simulink model "Smart_Grid_2"  (R2024b)
settings: Solver=FixedStepAuto  StartTime=0.0  StopTime=0.5  FixedStep=1e-5  RelTol=1e-3
undefined symbols (not defined in the file): Ion, Lithium
libraries: spsSeriesRLCBranchLib x76, spsRMSLib x65, spsIGBTDiodeLib x41, eeGeneralControl x36, slpidlib x34, spsThreePhaseVIMeasurementLib x32, spsVoltageMeasurementLib x18, simulink x16, spsCurrentMeasurementLib x15, spsThreePhaseBreakerLib x12, spsAlphaBetaZerotodq0Lib x12, spsPower3phPhasorLib x10
(part 7 of 8)

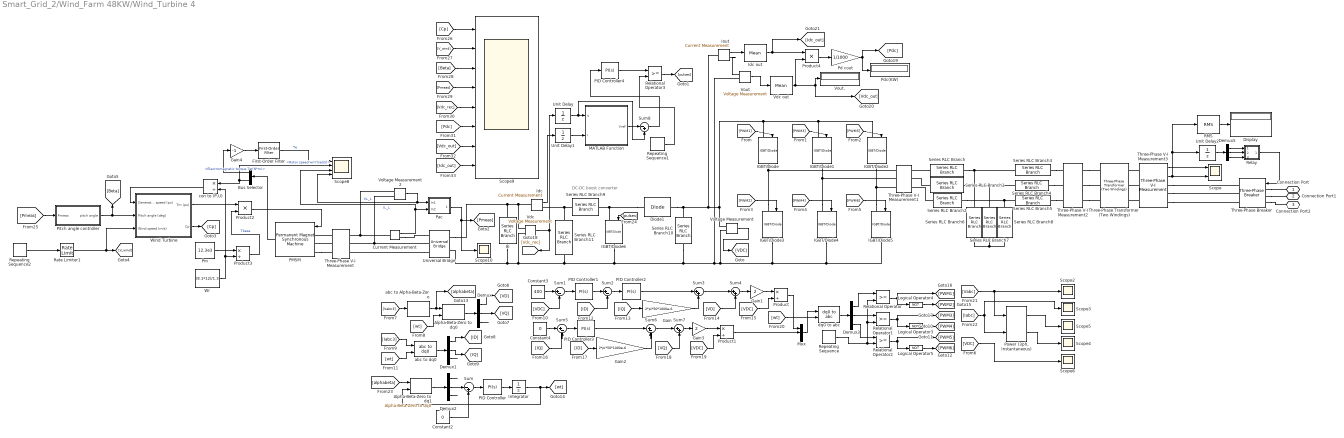
== system Smart_Grid_2/Wind_Farm 48KW/Wind_Turbine 4 ==
  note: DC-DC boost converter
  Alpha-Beta-Zero to dq0 : spsAlphaBetaZerotodq0Lib/Alpha-Beta-Zero to dq0  Alignment=90 degrees behind phase A axis
  Alpha-Beta-Zero to dq1 : spsAlphaBetaZerotodq0Lib/Alpha-Beta-Zero to dq0  Alignment=90 degrees behind phase A axis
  Bus Selector : BusSelector  OutputSignals=Electromagnetic torque Te (N*m),Rotor speed wm (rad/s)
  Ci : spsSeriesRLCBranchLib/Series RLC Branch  LConnTagsString=__new0  RConnTagsString=__new0  BranchType=RC  Resistance=0.005  Inductance=1e-3  SetiL0=off  InitialCurrent=0  Capacitance=500e-6  Setx0=off  InitialVoltage=0  Measurements=None
  Constant2 : Constant  Value=0
  Constant3 : Constant  Value=400
  Constant4 : Constant  Value=0
  Current Measurement : spsCurrentMeasurementLib/Current Measurement  PhasorSimulation=off  OutputType=Complex  PSBequivalent=0
  Demux{,1..3,5} (5 alike) : Demux  Outputs=3
  Diode1 : spsDiodeLib/Diode  Ron=0.001  Lon=0  Vf=0.8  IC=0  UseSnubber=0  Rs=500  Cs=250e-9  Measurements=off
  Display : Display
  First-Order Filter : spsFirstOrderFilterLib/First-Order Filter  FilterType=Lowpass  Tc=10e-3  Ts=50e-6  Initialize=on  Vac_Init=[0, 0, 50]  Vdc_Init=0  PlotResponse=off  FreqRange="[0,  200,  1]"
  Gain : Gain  Gain=2*pi*50*1000e-6
  Gain1 : Gain  Gain=2
  Gain2 : Gain  Gain=2*pi*50*1000e-6
  Gain3 : Gain  Gain=2
  Gain4 : Gain  Gain=-1
  IGBT/Diode{,1..6} (7 alike) : spsIGBTDiodeLib/IGBT//Diode  Ron=1e-3  Rs=1e5  Cs=inf  Measurements=off
  Idc : spsCurrentMeasurementLib/Current Measurement  PhasorSimulation=off  OutputType=Complex  PSBequivalent=0
  Idc out : spsMeanLib/Mean  Freq=50  Vinit=0  Ts=50e-6
  Integrator : Integrator
  Iout : spsCurrentMeasurementLib/Current Measurement  PhasorSimulation=off  OutputType=Complex  PSBequivalent=0
  Logical Operator3 : Logic  Operator=NOT  AllPortsSameDT=off  OutDataTypeStr=boolean
  Logical Operator4 : Logic  Operator=NOT  AllPortsSameDT=off  OutDataTypeStr=boolean
  Logical Operator5 : Logic  Operator=NOT  AllPortsSameDT=off  OutDataTypeStr=boolean
  MATLAB Function : MATLAB Function  TreatAsAtomicUnit=on
  Mux : Mux  Inputs=3
  PID Controller : slpidlib/PID Controller  Controller=PI  Form=Parallel  TimeDomain=Continuous-time  UseExternalTs=off  SampleTime=-1  IntegratorMethod=Forward Euler  FilterMethod=Forward Euler  ControllerParametersSource=internal  P=10  I=50000  UseKiTs=off  D=0  UseExternalDerivativeSource=off  N=100  UseFilter=on  TunerSelectOption=Transfer Function Based (PID Tuner App)  InitialConditionSource=internal  InitialConditionForIntegrator=0  InitialConditionForFilter=0  DifferentiatorICPrevScaledInput=0  ExternalReset=none  TrackingMode=off  Kt=1  LimitOutput=off  SatLimitsSource=internal  UpperSaturationLimit=inf  LowerSaturationLimit=-inf  LinearizeAsGain=on  AntiWindupMode=none  Kb=1  LimitIntegrator=off  UpperIntegratorSaturationLimit=inf  LowerIntegratorSaturationLimit=-inf  POutMin=[]  POutMax=[]  IOutMin=[]  IOutMax=[]  DOutMin=[]  DOutMax=[]  NOutMin=[]  NOutMax=[]  SumOutMin=[]  SumOutMax=[]  SaturationOutMin=[]  SaturationOutMax=[]  PParamMin=[]  PParamMax=[]  IParamMin=[]  IParamMax=[]  DParamMin=[]  DParamMax=[]  NParamMin=[]  NParamMax=[]  KbParamMin=[]  KbParamMax=[]  KtParamMin=[]  KtParamMax=[]  KbOutMin=[]  KbOutMax=[]  KtOutMin=[]  KtOutMax=[]  IntegratorOutMin=[]  IntegratorOutMax=[]  FilterOutMin=[]  FilterOutMax=[]  SumI1OutMin=[]  SumI1OutMax=[]  SumI2OutMin=[]  SumI2OutMax=[]  SumI3OutMin=[]  SumI3OutMax=[]  SumI4OutMin=[]  SumI4OutMax=[]  SumDOutMin=[]  SumDOutMax=[]  DifferentiatorOutMin=[]  DifferentiatorOutMax=[]  FilterDiffOutCoefMin=[]  FilterDiffOutCoefMax=[]  ReciprocalOutMin=[]  ReciprocalOutMax=[]  SumDenOutMin=[]  SumDenOutMax=[]  SumNumOutMin=[]  SumNumOutMax=[]  DivideOutMin=[]  DivideOutMax=[]  UdiffTsProdOutMin=[]  UdiffTsProdOutMax=[]  NTsProdOutMin=[]  NTsProdOutMax=[]  UintegralTsProdOutMin=[]  UintegralTsProdOutMax=[]  UngainTsProdOutMin=[]  UngainTsProdOutMax=[]  ClampingZeroOutDataTypeStr=Inherit: Inherit via back propagation  ClampingZeroOutMin=[]  ClampingZeroOutMax=[]  FilterDenConstantOutDataTypeStr=Inherit: Inherit via back propagation  FilterDenConstantOutMin=[]  FilterDenConstantOutMax=[]  PCopyOutDataTypeStr=Inherit: Inherit via back propagation  PCopyOutMin=[]  PCopyOutMax=[]  NCopyOutDataTypeStr=Inherit: Inherit via back propagation  NCopyOutMin=[]  NCopyOutMax=[]  IntegratorContinuousStateAttributes=''  IntegratorStateMustResolveToSignalObject=off  IntegratorRTWStateStorageClass=Auto  FilterContinuousStateAttributes=''  FilterStateMustResolveToSignalObject=off  FilterRTWStateStorageClass=Auto  ParallelPVariant=InternalParameters  IdealPVariant=Disabled  IVariant=InternalParameters  DVariant=Disabled  IntegratorVariant=Continuous  SatVariant=Disabled  AWVariant=Passthrough  PCopyVariant=Disabled  TRVariant=Disabled  FdbkBlocksVariant=Forward  IdealPFdbkVariant=Disabled  SatFdbkVariant=Disabled  DerivativeFilterVariant=Disabled  NVariant=Disabled  NCopyVariant=Disabled_SignalSpec  FilterICVariant=Disabled  IntegratorICVariant=InternalICs  ExternalResetVariant=Disabled  TRSumVariant=Passthrough  SumFdbkVariant=Disabled  SumVariant=Sum_PI  TsampFilterVariant=InternalTs  TsampNgainVariant=Passthrough  TsampIntegralVariant=Disabled_SignalSpec  ExternalSaturationOutDataTypeStr=Inherit: Same as second input  DerivativeSourceVariant=Disabled  PreIntVariant=InternalPreInt
  PID Controller1 : slpidlib/PID Controller  Controller=PI  Form=Parallel  TimeDomain=Continuous-time  UseExternalTs=off  SampleTime=-1  IntegratorMethod=Forward Euler  FilterMethod=Forward Euler  ControllerParametersSource=internal  P=0.25  I=300  UseKiTs=off  D=0  UseExternalDerivativeSource=off  N=100  UseFilter=on  TunerSelectOption=Transfer Function Based (PID Tuner App)  InitialConditionSource=internal  InitialConditionForIntegrator=0  InitialConditionForFilter=0  DifferentiatorICPrevScaledInput=0  ExternalReset=none  TrackingMode=off  Kt=1  LimitOutput=off  SatLimitsSource=internal  UpperSaturationLimit=inf  LowerSaturationLimit=-inf  LinearizeAsGain=on  AntiWindupMode=none  Kb=1  LimitIntegrator=off  UpperIntegratorSaturationLimit=inf  LowerIntegratorSaturationLimit=-inf  POutMin=[]  POutMax=[]  IOutMin=[]  IOutMax=[]  DOutMin=[]  DOutMax=[]  NOutMin=[]  NOutMax=[]  SumOutMin=[]  SumOutMax=[]  SaturationOutMin=[]  SaturationOutMax=[]  PParamMin=[]  PParamMax=[]  IParamMin=[]  IParamMax=[]  DParamMin=[]  DParamMax=[]  NParamMin=[]  NParamMax=[]  KbParamMin=[]  KbParamMax=[]  KtParamMin=[]  KtParamMax=[]  KbOutMin=[]  KbOutMax=[]  KtOutMin=[]  KtOutMax=[]  IntegratorOutMin=[]  IntegratorOutMax=[]  FilterOutMin=[]  FilterOutMax=[]  SumI1OutMin=[]  SumI1OutMax=[]  SumI2OutMin=[]  SumI2OutMax=[]  SumI3OutMin=[]  SumI3OutMax=[]  SumI4OutMin=[]  SumI4OutMax=[]  SumDOutMin=[]  SumDOutMax=[]  DifferentiatorOutMin=[]  DifferentiatorOutMax=[]  FilterDiffOutCoefMin=[]  FilterDiffOutCoefMax=[]  ReciprocalOutMin=[]  ReciprocalOutMax=[]  SumDenOutMin=[]  SumDenOutMax=[]  SumNumOutMin=[]  SumNumOutMax=[]  DivideOutMin=[]  DivideOutMax=[]  UdiffTsProdOutMin=[]  UdiffTsProdOutMax=[]  NTsProdOutMin=[]  NTsProdOutMax=[]  UintegralTsProdOutMin=[]  UintegralTsProdOutMax=[]  UngainTsProdOutMin=[]  UngainTsProdOutMax=[]  ClampingZeroOutDataTypeStr=Inherit: Inherit via back propagation  ClampingZeroOutMin=[]  ClampingZeroOutMax=[]  FilterDenConstantOutDataTypeStr=Inherit: Inherit via back propagation  FilterDenConstantOutMin=[]  FilterDenConstantOutMax=[]  PCopyOutDataTypeStr=Inherit: Inherit via back propagation  PCopyOutMin=[]  PCopyOutMax=[]  NCopyOutDataTypeStr=Inherit: Inherit via back propagation  NCopyOutMin=[]  NCopyOutMax=[]  IntegratorContinuousStateAttributes=''  IntegratorStateMustResolveToSignalObject=off  IntegratorRTWStateStorageClass=Auto  FilterContinuousStateAttributes=''  FilterStateMustResolveToSignalObject=off  FilterRTWStateStorageClass=Auto  ParallelPVariant=InternalParameters  IdealPVariant=Disabled  IVariant=InternalParameters  DVariant=Disabled  IntegratorVariant=Continuous  SatVariant=Disabled  AWVariant=Passthrough  PCopyVariant=Disabled  TRVariant=Disabled  FdbkBlocksVariant=Forward  IdealPFdbkVariant=Disabled  SatFdbkVariant=Disabled  DerivativeFilterVariant=Disabled  NVariant=Disabled  NCopyVariant=Disabled_SignalSpec  FilterICVariant=Disabled  IntegratorICVariant=InternalICs  ExternalResetVariant=Disabled  TRSumVariant=Passthrough  SumFdbkVariant=Disabled  SumVariant=Sum_PI  TsampFilterVariant=InternalTs  TsampNgainVariant=Passthrough  TsampIntegralVariant=Disabled_SignalSpec  ExternalSaturationOutDataTypeStr=Inherit: Same as second input  DerivativeSourceVariant=Disabled  PreIntVariant=InternalPreInt
  PID Controller2 : slpidlib/PID Controller  Controller=PI  Form=Parallel  TimeDomain=Continuous-time  UseExternalTs=off  SampleTime=-1  IntegratorMethod=Forward Euler  FilterMethod=Forward Euler  ControllerParametersSource=internal  P=10  I=20  UseKiTs=off  D=0  UseExternalDerivativeSource=off  N=100  UseFilter=on  TunerSelectOption=Transfer Function Based (PID Tuner App)  InitialConditionSource=internal  InitialConditionForIntegrator=0  InitialConditionForFilter=0  DifferentiatorICPrevScaledInput=0  ExternalReset=none  TrackingMode=off  Kt=1  LimitOutput=off  SatLimitsSource=internal  UpperSaturationLimit=inf  LowerSaturationLimit=-inf  LinearizeAsGain=on  AntiWindupMode=none  Kb=1  LimitIntegrator=off  UpperIntegratorSaturationLimit=inf  LowerIntegratorSaturationLimit=-inf  POutMin=[]  POutMax=[]  IOutMin=[]  IOutMax=[]  DOutMin=[]  DOutMax=[]  NOutMin=[]  NOutMax=[]  SumOutMin=[]  SumOutMax=[]  SaturationOutMin=[]  SaturationOutMax=[]  PParamMin=[]  PParamMax=[]  IParamMin=[]  IParamMax=[]  DParamMin=[]  DParamMax=[]  NParamMin=[]  NParamMax=[]  KbParamMin=[]  KbParamMax=[]  KtParamMin=[]  KtParamMax=[]  KbOutMin=[]  KbOutMax=[]  KtOutMin=[]  KtOutMax=[]  IntegratorOutMin=[]  IntegratorOutMax=[]  FilterOutMin=[]  FilterOutMax=[]  SumI1OutMin=[]  SumI1OutMax=[]  SumI2OutMin=[]  SumI2OutMax=[]  SumI3OutMin=[]  SumI3OutMax=[]  SumI4OutMin=[]  SumI4OutMax=[]  SumDOutMin=[]  SumDOutMax=[]  DifferentiatorOutMin=[]  DifferentiatorOutMax=[]  FilterDiffOutCoefMin=[]  FilterDiffOutCoefMax=[]  ReciprocalOutMin=[]  ReciprocalOutMax=[]  SumDenOutMin=[]  SumDenOutMax=[]  SumNumOutMin=[]  SumNumOutMax=[]  DivideOutMin=[]  DivideOutMax=[]  UdiffTsProdOutMin=[]  UdiffTsProdOutMax=[]  NTsProdOutMin=[]  NTsProdOutMax=[]  UintegralTsProdOutMin=[]  UintegralTsProdOutMax=[]  UngainTsProdOutMin=[]  UngainTsProdOutMax=[]  ClampingZeroOutDataTypeStr=Inherit: Inherit via back propagation  ClampingZeroOutMin=[]  ClampingZeroOutMax=[]  FilterDenConstantOutDataTypeStr=Inherit: Inherit via back propagation  FilterDenConstantOutMin=[]  FilterDenConstantOutMax=[]  PCopyOutDataTypeStr=Inherit: Inherit via back propagation  PCopyOutMin=[]  PCopyOutMax=[]  NCopyOutDataTypeStr=Inherit: Inherit via back propagation  NCopyOutMin=[]  NCopyOutMax=[]  IntegratorContinuousStateAttributes=''  IntegratorStateMustResolveToSignalObject=off  IntegratorRTWStateStorageClass=Auto  FilterContinuousStateAttributes=''  FilterStateMustResolveToSignalObject=off  FilterRTWStateStorageClass=Auto  ParallelPVariant=InternalParameters  IdealPVariant=Disabled  IVariant=InternalParameters  DVariant=Disabled  IntegratorVariant=Continuous  SatVariant=Disabled  AWVariant=Passthrough  PCopyVariant=Disabled  TRVariant=Disabled  FdbkBlocksVariant=Forward  IdealPFdbkVariant=Disabled  SatFdbkVariant=Disabled  DerivativeFilterVariant=Disabled  NVariant=Disabled  NCopyVariant=Disabled_SignalSpec  FilterICVariant=Disabled  IntegratorICVariant=InternalICs  ExternalResetVariant=Disabled  TRSumVariant=Passthrough  SumFdbkVariant=Disabled  SumVariant=Sum_PI  TsampFilterVariant=InternalTs  TsampNgainVariant=Passthrough  TsampIntegralVariant=Disabled_SignalSpec  ExternalSaturationOutDataTypeStr=Inherit: Same as second input  DerivativeSourceVariant=Disabled  PreIntVariant=InternalPreInt
  PID Controller3 : slpidlib/PID Controller  Controller=PI  Form=Parallel  TimeDomain=Continuous-time  UseExternalTs=off  SampleTime=-1  IntegratorMethod=Forward Euler  FilterMethod=Forward Euler  ControllerParametersSource=internal  P=10  I=20  UseKiTs=off  D=0  UseExternalDerivativeSource=off  N=100  UseFilter=on  TunerSelectOption=Transfer Function Based (PID Tuner App)  InitialConditionSource=internal  InitialConditionForIntegrator=0  InitialConditionForFilter=0  DifferentiatorICPrevScaledInput=0  ExternalReset=none  TrackingMode=off  Kt=1  LimitOutput=off  SatLimitsSource=internal  UpperSaturationLimit=inf  LowerSaturationLimit=-inf  LinearizeAsGain=on  AntiWindupMode=none  Kb=1  LimitIntegrator=off  UpperIntegratorSaturationLimit=inf  LowerIntegratorSaturationLimit=-inf  POutMin=[]  POutMax=[]  IOutMin=[]  IOutMax=[]  DOutMin=[]  DOutMax=[]  NOutMin=[]  NOutMax=[]  SumOutMin=[]  SumOutMax=[]  SaturationOutMin=[]  SaturationOutMax=[]  PParamMin=[]  PParamMax=[]  IParamMin=[]  IParamMax=[]  DParamMin=[]  DParamMax=[]  NParamMin=[]  NParamMax=[]  KbParamMin=[]  KbParamMax=[]  KtParamMin=[]  KtParamMax=[]  KbOutMin=[]  KbOutMax=[]  KtOutMin=[]  KtOutMax=[]  IntegratorOutMin=[]  IntegratorOutMax=[]  FilterOutMin=[]  FilterOutMax=[]  SumI1OutMin=[]  SumI1OutMax=[]  SumI2OutMin=[]  SumI2OutMax=[]  SumI3OutMin=[]  SumI3OutMax=[]  SumI4OutMin=[]  SumI4OutMax=[]  SumDOutMin=[]  SumDOutMax=[]  DifferentiatorOutMin=[]  DifferentiatorOutMax=[]  FilterDiffOutCoefMin=[]  FilterDiffOutCoefMax=[]  ReciprocalOutMin=[]  ReciprocalOutMax=[]  SumDenOutMin=[]  SumDenOutMax=[]  SumNumOutMin=[]  SumNumOutMax=[]  DivideOutMin=[]  DivideOutMax=[]  UdiffTsProdOutMin=[]  UdiffTsProdOutMax=[]  NTsProdOutMin=[]  NTsProdOutMax=[]  UintegralTsProdOutMin=[]  UintegralTsProdOutMax=[]  UngainTsProdOutMin=[]  UngainTsProdOutMax=[]  ClampingZeroOutDataTypeStr=Inherit: Inherit via back propagation  ClampingZeroOutMin=[]  ClampingZeroOutMax=[]  FilterDenConstantOutDataTypeStr=Inherit: Inherit via back propagation  FilterDenConstantOutMin=[]  FilterDenConstantOutMax=[]  PCopyOutDataTypeStr=Inherit: Inherit via back propagation  PCopyOutMin=[]  PCopyOutMax=[]  NCopyOutDataTypeStr=Inherit: Inherit via back propagation  NCopyOutMin=[]  NCopyOutMax=[]  IntegratorContinuousStateAttributes=''  IntegratorStateMustResolveToSignalObject=off  IntegratorRTWStateStorageClass=Auto  FilterContinuousStateAttributes=''  FilterStateMustResolveToSignalObject=off  FilterRTWStateStorageClass=Auto  ParallelPVariant=InternalParameters  IdealPVariant=Disabled  IVariant=InternalParameters  DVariant=Disabled  IntegratorVariant=Continuous  SatVariant=Disabled  AWVariant=Passthrough  PCopyVariant=Disabled  TRVariant=Disabled  FdbkBlocksVariant=Forward  IdealPFdbkVariant=Disabled  SatFdbkVariant=Disabled  DerivativeFilterVariant=Disabled  NVariant=Disabled  NCopyVariant=Disabled_SignalSpec  FilterICVariant=Disabled  IntegratorICVariant=InternalICs  ExternalResetVariant=Disabled  TRSumVariant=Passthrough  SumFdbkVariant=Disabled  SumVariant=Sum_PI  TsampFilterVariant=InternalTs  TsampNgainVariant=Passthrough  TsampIntegralVariant=Disabled_SignalSpec  ExternalSaturationOutDataTypeStr=Inherit: Same as second input  DerivativeSourceVariant=Disabled  PreIntVariant=InternalPreInt
  PID Controller4 : slpidlib/PID Controller  Controller=PI  Form=Parallel  TimeDomain=Continuous-time  UseExternalTs=off  SampleTime=-1  IntegratorMethod=Forward Euler  FilterMethod=Forward Euler  ControllerParametersSource=internal  P=0.005  I=0.001  UseKiTs=off  D=0  UseExternalDerivativeSource=off  N=100  UseFilter=on  TunerSelectOption=Transfer Function Based (PID Tuner App)  InitialConditionSource=internal  InitialConditionForIntegrator=0  InitialConditionForFilter=0  DifferentiatorICPrevScaledInput=0  ExternalReset=none  TrackingMode=off  Kt=1  LimitOutput=on  SatLimitsSource=internal  UpperSaturationLimit=0.95  LowerSaturationLimit=0  LinearizeAsGain=on  AntiWindupMode=none  Kb=1  LimitIntegrator=off  UpperIntegratorSaturationLimit=inf  LowerIntegratorSaturationLimit=-inf  POutMin=[]  POutMax=[]  IOutMin=[]  IOutMax=[]  DOutMin=[]  DOutMax=[]  NOutMin=[]  NOutMax=[]  SumOutMin=[]  SumOutMax=[]  SaturationOutMin=[]  SaturationOutMax=[]  PParamMin=[]  PParamMax=[]  IParamMin=[]  IParamMax=[]  DParamMin=[]  DParamMax=[]  NParamMin=[]  NParamMax=[]  KbParamMin=[]  KbParamMax=[]  KtParamMin=[]  KtParamMax=[]  KbOutMin=[]  KbOutMax=[]  KtOutMin=[]  KtOutMax=[]  IntegratorOutMin=[]  IntegratorOutMax=[]  FilterOutMin=[]  FilterOutMax=[]  SumI1OutMin=[]  SumI1OutMax=[]  SumI2OutMin=[]  SumI2OutMax=[]  SumI3OutMin=[]  SumI3OutMax=[]  SumI4OutMin=[]  SumI4OutMax=[]  SumDOutMin=[]  SumDOutMax=[]  DifferentiatorOutMin=[]  DifferentiatorOutMax=[]  FilterDiffOutCoefMin=[]  FilterDiffOutCoefMax=[]  ReciprocalOutMin=[]  ReciprocalOutMax=[]  SumDenOutMin=[]  SumDenOutMax=[]  SumNumOutMin=[]  SumNumOutMax=[]  DivideOutMin=[]  DivideOutMax=[]  UdiffTsProdOutMin=[]  UdiffTsProdOutMax=[]  NTsProdOutMin=[]  NTsProdOutMax=[]  UintegralTsProdOutMin=[]  UintegralTsProdOutMax=[]  UngainTsProdOutMin=[]  UngainTsProdOutMax=[]  ClampingZeroOutDataTypeStr=Inherit: Inherit via back propagation  ClampingZeroOutMin=[]  ClampingZeroOutMax=[]  FilterDenConstantOutDataTypeStr=Inherit: Inherit via back propagation  FilterDenConstantOutMin=[]  FilterDenConstantOutMax=[]  PCopyOutDataTypeStr=Inherit: Inherit via back propagation  PCopyOutMin=[]  PCopyOutMax=[]  NCopyOutDataTypeStr=Inherit: Inherit via back propagation  NCopyOutMin=[]  NCopyOutMax=[]  IntegratorContinuousStateAttributes=''  IntegratorStateMustResolveToSignalObject=off  IntegratorRTWStateStorageClass=Auto  FilterContinuousStateAttributes=''  FilterStateMustResolveToSignalObject=off  FilterRTWStateStorageClass=Auto  ParallelPVariant=InternalParameters  IdealPVariant=Disabled  IVariant=InternalParameters  DVariant=Disabled  IntegratorVariant=Continuous  SatVariant=Enabled  AWVariant=Passthrough  PCopyVariant=Disabled  TRVariant=Disabled  FdbkBlocksVariant=Forward  IdealPFdbkVariant=Disabled  SatFdbkVariant=Disabled  DerivativeFilterVariant=Disabled  NVariant=Disabled  NCopyVariant=Disabled_SignalSpec  FilterICVariant=Disabled  IntegratorICVariant=InternalICs  ExternalResetVariant=Disabled  TRSumVariant=Passthrough  SumFdbkVariant=Disabled  SumVariant=Sum_PI  TsampFilterVariant=InternalTs  TsampNgainVariant=Passthrough  TsampIntegralVariant=Disabled_SignalSpec  ExternalSaturationOutDataTypeStr=Inherit: Same as second input  DerivativeSourceVariant=Disabled  PreIntVariant=InternalPreInt
  PMSM : spsPermanentMagnetSynchronousMachineLib/Permanent Magnet Synchronous Machine  NbPhases=3  FluxDistribution=Sinusoidal  RotorType=Salient-pole  MechanicalLoad=Torque Tm  PresetModel=No  ShowDetailedParameters=on  MeasurementBus=off  Resistance=0.0485  Inductance=8.5e-3  dqInductances=[0.395e-3,0.395e-3]  La=0.000395  MachineConstant=Flux linkage established by magnets (V.s)  Flux=0.1194  VoltageCst=86.6271  TorqueCst=0.7164  Flat=120  Mechanical=[0.0027 0.0004924 4 0]  PolePairs=4  InitialConditions=[0,0, 0,0]  InitialConditions5ph=[0 0 0 0 0 0]  RefAngle=90 degrees behind phase A axis (modified Park)  IterativeDiscreteModel=Trapezoidal non iterative  TsBlock=-1  TsPowergui=0
  Pac : Subsystem
  Pd cout : Gain  Gain=1/1000
  Pdc(KW) : Display
  "Pitch angle controller " : Subsystem
  Pm : Constant  Value=12.3e3
  "Power (3ph, Instantaneous)" : spsPower3phInstantaneousLib/Power (3ph, Instantaneous)
  Product : Product  Inputs=*/
  Product1 : Product  Inputs=*/
  Product2 : Product  Inputs=**
  Product3 : Product  Inputs=*/
  Product4 : Product
  RMS : spsRMSLib/RMS  TrueRMS=on  Freq=50  RMSInit=0  Ts=0.001
  Rate Limiter1 : RateLimiter  RisingSlewLimit=5  FallingSlewLimit=-5  SampleTimeMode=inherited  InitialCondition=12
  Relational Operator{,1..3} (4 alike) : RelationalOperator  OutDataTypeStr=boolean  RndMeth=Simplest  InputSameDT=off
  Relay : Subsystem
  Repeating Sequence : simulink/Sources/Repeating Sequence  rep_seq_t=[0 0.00005 0.0001]  rep_seq_y=[-1 1 -1]
  Repeating Sequence1 : simulink/Sources/Repeating Sequence  rep_seq_t=[0 0.0002]  rep_seq_y=[0 1]
  Repeating Sequence2 : simulink/Sources/Repeating Sequence  rep_seq_t=|  rep_seq_y=|
      rep_seq_t=|
      | [0
      | 0.050505051
      | 0.101010101
      | 0.151515152
      | 0.202020202
      | 0.252525253
      | 0.303030303
      | 0.353535354
      | 0.404040404
      | 0.454545455
      | 0.505050505
      | 0.555555556
      | 0.606060606
      | 0.656565657
      | 0.707070707
      | 0.757575758
      | 0.808080808
      | 0.858585859
      | 0.909090909
      | 0.95959596
      | 1.01010101
      | 1.060606061
      | 1.111111111
      | 1.161616162
      | 1.212121212
      | 1.262626263
      | 1.313131313
      | 1.363636364
      | 1.414141414
      | 1.464646465
      | 1.515151515
      | 1.565656566
      | 1.616161616
      | 1.666666667
      | 1.717171717
      | 1.767676768
      | 1.818181818
      | 1.868686869
      | 1.919191919
      | 1.96969697
      | 2.02020202
      | 2.070707071
      | 2.121212121
      | 2.171717172
      | 2.222222222
      | 2.272727273
      | 2.323232323
      | 2.373737374
      | 2.424242424
      | 2.474747475
      | 2.525252525
      | 2.575757576
      | 2.626262626
      | 2.676767677
      | 2.727272727
      | 2.777777778
      | 2.828282828
      | 2.878787879
      | 2.929292929
      | 2.97979798
      | 3.03030303
      | 3.080808081
      | 3.131313131
      | 3.181818182
      | 3.232323232
      | 3.282828283
      | 3.333333333
      | 3.383838384
      | 3.434343434
      | 3.484848485
      | 3.535353535
      | 3.585858586
      | 3.636363636
      | 3.686868687
      | 3.737373737
      | 3.787878788
      | 3.838383838
      | 3.888888889
      | 3.939393939
      | 3.98989899
      | 4.04040404
      | 4.090909091
      | 4.141414141
      | 4.191919192
      | 4.242424242
      | 4.292929293
      | 4.343434343
      | 4.393939394
      | 4.444444444
      | 4.494949495
      | 4.545454545
      | 4.595959596
      | 4.646464646
      | 4.696969697
      | 4.747474747
      | 4.797979798
      | 4.848484848
      | 4.898989899
      | 4.949494949
      | 5
      | ]
      rep_seq_y=|
      | [11.28656082
      | 8.455585009
      | 10.96465173
      | 12.63991376
      | 12.63418909
      | 13.43810467
      | 11.23402126
      | 9.2084575
      | 9.597895253
      | 13.38497279
      | 13.84766295
      | 9.012729612
      | 8.284144965
      | 9.838713946
      | 14.70035396
      | 9.912390412
      | 11.28086829
      | 9.783668071
      | 9.931481374
      | 11.37307541
      | 13.31473417
      | 8.526985036
      | 13.85182887
      | 14.59275739
      | 8.380161753
      | 9.958960128
      | 8.702886747
      | 14.27173227
      | 8.102779683
      | 10.4076636
      | 14.44876127
      | 8.300229502
      | 13.37218818
      | 11.12358601
      | 13.58944894
      | 8.394933897
      | 13.57404909
      | 13.1032934
      | 12.96110812
      | 11.61975924
      | 12.47155544
      | 10.77994608
      | 12.06075426
      | 13.38886857
      | 13.17758286
      | 13.21186929
      | 8.671134656
      | 13.75397495
      | 10.29202347
      | 8.290332305
      | 11.89873046
      | 14.58902826
      | 10.52581478
      | 9.926313109
      | 14.25001594
      | 11.67947423
      | 11.01487597
      | 10.1796175
      | 11.29988996
      | 12.98527552
      | 9.579685971
      | 8.030683641
      | 9.300667004
      | 12.77961401
      | 13.38525952
      | 10.19829
      | 13.36479246
      | 13.57819968
      | 9.836912603
      | 14.11393522
      | 8.481542733
      | 0
      | 0
      | 0
      | 0
      | 0
      | 0
      | 8.231879915
      | 9.829213716
      | 10.68985499
      | 9.755757856
      | 13.79545802
      | 9.097755566
      | 12.81065629
      | 9.93242825
      | 10.95840187
      | 9.395979639
      | 14.14661616
      | 10.27824804
      | 11.81440015
      | 14.38877705
      | 11.1968821
      | 13.15702571
      | 13.53194587
      | 12.5149219
      | 13.65086698
      | 11.70877998
      | 9.68709541
      | 12.0944941
      | 14.41275822
      | ]
  Scope : Scope  NumInputPorts=2
  Scope{2..6,10} (6 alike) : Scope
  Scope8 : Scope  NumInputPorts=4
  Scope9 : Scope  NumInputPorts=8
  Series RLC Branch{,1..5} (6 alike) : spsSeriesRLCBranchLib/Series RLC Branch  LConnTagsString=__new0  RConnTagsString=__new0  BranchType=RL  Resistance=1e-6  Inductance=2.32e-3  SetiL0=off  InitialCurrent=0  Capacitance=1e-6  Setx0=off  InitialVoltage=0  Measurements=None
  Series RLC Branch10 : spsSeriesRLCBranchLib/Series RLC Branch  LConnTagsString=__new0  RConnTagsString=__new0  BranchType=RC  Resistance=0.005  Inductance=1e-3  SetiL0=off  InitialCurrent=0  Capacitance=6.6094e-04  Setx0=off  InitialVoltage=0  Measurements=None
  Series RLC Branch11 : spsSeriesRLCBranchLib/Series RLC Branch  LConnTagsString=__new0  RConnTagsString=__new0  BranchType=RC  Resistance=1e-3  Inductance=1e-3  SetiL0=off  InitialCurrent=0  Capacitance=100e-6  Setx0=off  InitialVoltage=0  Measurements=None
  Series RLC Branch6 : spsSeriesRLCBranchLib/Series RLC Branch  LConnTagsString=__new0  RConnTagsString=__new0  BranchType=RC  Resistance=1e-6  Inductance=500e-6  SetiL0=off  InitialCurrent=0  Capacitance=9.37e-6  Setx0=off  InitialVoltage=0  Measurements=None
  Series RLC Branch7 : spsSeriesRLCBranchLib/Series RLC Branch  LConnTagsString=__new0  RConnTagsString=__new0  BranchType=RC  Resistance=1e-6  Inductance=500e-6  SetiL0=off  InitialCurrent=0  Capacitance=9.37e-6  Setx0=off  InitialVoltage=0  Measurements=None
  Series RLC Branch8 : spsSeriesRLCBranchLib/Series RLC Branch  LConnTagsString=__new0  RConnTagsString=__new0  BranchType=RC  Resistance=1e-6  Inductance=500e-6  SetiL0=off  InitialCurrent=0  Capacitance=9.37e-6  Setx0=off  InitialVoltage=0  Measurements=None
  Series RLC Branch9 : spsSeriesRLCBranchLib/Series RLC Branch  LConnTagsString=__new0  RConnTagsString=__new0  BranchType=L  Resistance=0.005  Inductance=4.5573e-05  SetiL0=off  InitialCurrent=0  Capacitance=500e-6  Setx0=off  InitialVoltage=0  Measurements=None
  Sum : Sum  Inputs=|-+
  Sum{1..2,5..6} (4 alike) : Sum  Inputs=|+-
  Sum3 : Sum  Inputs=|++
  Sum4 : Sum  Inputs=|++
  Sum7 : Sum  Inputs=|++
  Sum8 : Sum  Inputs=|-+
  Three-Phase Transformer (Two Windings) : spsThreePhaseTransformerTwoWindingsLib/Three-Phase Transformer (Two Windings)  Winding1Connection=Yg  Winding2Connection=Yg  CoreType=Three single-phase transformers  SetSaturation=off  Hysteresis=off  DataFile='hysteresis'  SetInitialFlux=off  Measurements=None  UNITS=pu  NominalPower=[ 25e6 , 50 ]  Winding1=[ 400 , 0.002 , 0.08 ]  Winding2=[ 25e3 , 0.002 , 0.08 ]  Rm=500  Lm=500  L0=0.5  Saturation=[ 0,0 ; 0.0024,1.2 ; 1.0,1.52 ]  InitialFluxes=[ 0.8 , -0.8 , 0.7 ]  BreakLoop=off  DiscreteSolver=Trapezoidal iterative  DataType=off  TransfoNumber=1
  Three-Phase V-I Measurement : spsThreePhaseVIMeasurementLib/Three-Phase V-I Measurement  VoltageMeasurement=no  SetLabelV=off  LabelV=Vabc  Vpu=off  VpuLL=off  CurrentMeasurement=no  SetLabelI=off  LabelI=Iabc  Ipu=off  Pbase=100e6  Vbase=500e3  OutputType=Complex  PhasorSimulation=off  PSBequivalent=0
  Three-Phase V-I Measurement1 : spsThreePhaseVIMeasurementLib/Three-Phase V-I Measurement  VoltageMeasurement=no  SetLabelV=off  LabelV=Vabc  Vpu=off  VpuLL=off  CurrentMeasurement=yes  SetLabelI=on  LabelI=Iabc3  Ipu=off  Pbase=100e6  Vbase=500e3  OutputType=Complex  PhasorSimulation=off  PSBequivalent=0
  Three-Phase V-I Measurement2 : spsThreePhaseVIMeasurementLib/Three-Phase V-I Measurement  VoltageMeasurement=phase-to-ground  SetLabelV=on  LabelV=Vabc3  Vpu=off  VpuLL=off  CurrentMeasurement=no  SetLabelI=off  LabelI=Iabc  Ipu=off  Pbase=100e6  Vbase=500e3  OutputType=Complex  PhasorSimulation=off  PSBequivalent=0
  Three-Phase V-I Measurement3 : spsThreePhaseVIMeasurementLib/Three-Phase V-I Measurement  VoltageMeasurement=phase-to-ground  SetLabelV=off  LabelV=Vabc  Vpu=off  VpuLL=off  CurrentMeasurement=yes  SetLabelI=off  LabelI=Iabc  Ipu=off  Pbase=100e6  Vbase=500e3  OutputType=Complex  PhasorSimulation=off  PSBequivalent=0
  Three-Phase Breaker : spsThreePhaseBreakerLib/Three-Phase Breaker  InitialState=closed  SwitchA=on  SwitchB=on  SwitchC=on  SwitchTimes="[1/60  5/60]"  External=on  BreakerResistance=0.001  SnubberResistance=1e8  SnubberCapacitance=inf  Measurements=Breaker voltages and currents
  Unit Delay : UnitDelay  SampleTime=1e-4  HasFrameUpgradeWarning=on
  Unit Delay1 : UnitDelay  SampleTime=1e-4  HasFrameUpgradeWarning=on
  Unit Delay2 : UnitDelay  SampleTime=0.001  HasFrameUpgradeWarning=on
  Universal Bridge : spsUniversalBridgeLib/Universal Bridge  Arms=3  SnubberResistance=1e5  SnubberCapacitance=inf  Device=Diodes  Ron=1e-3  Lon=0  ForwardVoltages="[  0  0  ]"  ForwardVoltage=0  GTOparameters=[ 10e-6 , 20e-6 ]  IGBTparameters=[ 1e-6 , 2e-6 ]  Measurements=None  Measurements_2=None  converterType=Rectifier
  Vdc : spsVoltageMeasurementLib/Voltage Measurement  PhasorSimulation=off  OutputType=Complex  PSBequivalent=0
  Vdc out : spsMeanLib/Mean  Freq=50  Vinit=0  Ts=50e-6
  Voltage Measurement : spsVoltageMeasurementLib/Voltage Measurement  PhasorSimulation=off  OutputType=Complex  PSBequivalent=0
  Voltage Measurement2 : spsVoltageMeasurementLib/Voltage Measurement  PhasorSimulation=off  OutputType=Complex  PSBequivalent=0
  Vout : spsVoltageMeasurementLib/Voltage Measurement  PhasorSimulation=off  OutputType=Complex  PSBequivalent=0
  Vout. : Display
  Wind Turbine : Subsystem  AncestorBlock=sps_lib/Electrical Machines/Wind Turbine  DialogController=POWERSYS.PowerSysDialog  mask(Wind Turbine){Pnom=12.3e3, Pelec_base=12.3e3/0.9, wind_base=12, P_wind_base=0.85, speed_nom=1.2, pitch_angle=0, c1_c6=[0.51763          116          0.4            5           21     0.006795], cp_nom=0.48, lambda_nom=8.1}
      mask prompts: Pnom "Nominal mechanical output power (W):"; Pelec_base "Base power of the electrical generator (VA):"; wind_base "Base wind speed (m/s):"; P_wind_base "Maximum power at base wind speed (pu of nominal mechanical power):"; speed_nom "Base rotational speed (p.u. of base generator speed):"; pitch_angle "Pitch angle beta to display wind-turbine power characteristics (beta >=0)  (deg):"
      mask help:
      | This block implements a variable pitch wind turbine model. The performance coefficient Cp of the turbine is the mechanical output power of the turbine divided by wind power and a function of wind speed, rotational speed, and pitch angle (beta). Cp reaches its maximum value at zero beta. Select the wind-turbine power characteristics display to plot the turbine characteristics at the specified pitch angle.
      |
      | The first input is the generator speed in per unit of the generator base speed. For a synchronous or asynchronous generator, the base speed is the synchronous speed. For a permanent-magnet generator, the base speed is defined as the speed producing nominal voltage at  no load. The second input is the blade pitch angle (beta) in degrees. The third input is the wind speed in m/s.
      |
      | The output is the torque applied to the generator shaft in per unit of the generator ratings.
      |
      | The turbine inertia must be added to the generator inertia.
      mask init: same as Smart_Grid_2/Wind_Farm 48KW/Wind_Turbine 1/Wind Turbine
      settings: LibrarySourceBlock=sps_lib/Electrical Machines/Wind Turbine  OpenFcn=sps_rtmsupport('OpenFcn',gcbh)
      mask Help: helpview(psbhelp);
      mask DialogControl DisplayTurbChar Prompt: Display wind turbine power characteristics
      mask DialogControl DisplayTurbChar Callback: WindTurbinePlot(gcb)
  Wr : Constant  Value=(8.1*12)/1.3
  abc to Alpha-Beta-Zero : spsabctoAlphaBetaZeroLib/abc to Alpha-Beta-Zero
  abc to dq0 : spsabctodq0Lib/abc to dq0  Alignment=90 degrees behind phase A axis
  con to (P.U) : Product  Inputs=*/
  dq0 to abc : spsdq0toabcLib/dq0 to abc  Alignment=90 degrees behind phase A axis
  Connection Port : PMIOPort  Side=Right
  Connection Port1 : PMIOPort  Port=2  Side=Right
  Connection Port2 : PMIOPort  Port=3  Side=Right
  wires:
  Vdc/1 -> [Vdc_rec], Unit Delay/1
  Unit Delay1/1 -> MATLAB Function/2(I)
  Unit Delay/1 -> MATLAB Function/1(V), Sum8/2
  Sum8/1 -> PID Controller4/1
  PID Controller4/1 -> Relational Operator3/1
  Relational Operator3/1 -> [pulses]
  Idc/1 -> Unit Delay1/1
  Repeating Sequence1/1 -> Relational Operator3/2
  MATLAB Function/1(Vref) -> Sum8/1
  Rate Limiter1/1 -> Wind Turbine/3(Wind speed (m/s)), [V_wind]
  Demux/3 -> ?
  ? -> Mux/3
  Demux2/1 -> ?
  [V_wind] -> Scope9/2
  [Idc_out] -> Scope9/8
  [Vdc_out] -> Scope9/7
  [Beta] -> Scope9/3
  Pd cout/1 -> Pdc(KW)/1, [Pdc]
  Wind Turbine/2(Cp) -> [Cp]
  Gain4/1 -> First-Order Filter/1
  Bus Selector/1 -> Gain4/1  "<Electromagnetic torque Te (N*m)>"
  Product2/1 -> PMSM/1
  [Pmeas] -> "Pitch angle controller "/1(Pmeas)
  Current Measurement/1 -> Pac/2(In2), Scope8/3  "IL_L"
  PMSM/1 -> Bus Selector/1
  Pm/1 -> Product3/1
  con to (P.U)/1 -> Wind Turbine/1(Generator speed (pu))
  Product3/1 -> Product2/2  "Tbase"
  Wind Turbine/1(Tm (pu)) -> Product2/1
  First-Order Filter/1 -> Scope8/1  "Te"
  [pulses] -> IGBT/Diode6/1
  [Pdc] -> Scope9/6
  Product4/1 -> Pd cout/1
  Voltage Measurement/1 -> [VDC]
  [wt] -> Alpha-Beta-Zero to dq0/2
  Gain3/1 -> Product1/1
  Sum7/1 -> Gain3/1
  Mux/1 -> dq0 to abc/1
  [Cp] -> Scope9/1
  Gain/1 -> Sum3/2
  Relational Operator1/1 -> Logical Operator3/1, [PWM3]
  [Iabc3] -> abc to dq0/1
  Demux3/1 -> Relational Operator/1
  [VDC] -> Product/2
  Demux1/2 -> [IQ]
  [VDC] -> Sum1/2
  [Vabc] -> "Power (3ph, Instantaneous)"/1, Scope2/1
  Logical Operator5/1 -> [PWM6]
  [Vdc_rec] -> Scope9/5
  Constant3/1 -> Sum1/1
  Vout/1 -> Vdc out/1
  Demux2/2 -> Sum/1
  Sum6/1 -> Sum7/1
  [VDC] -> Product1/2
  [ID] -> Sum2/2
  [ID] -> Gain2/1
  Alpha-Beta-Zero to dq1/1 -> Demux2/1
  Idc out/1 -> [Idc_out], Product4/1
  [IQ] -> Gain/1
  Sum1/1 -> PID Controller1/1
  "Pitch angle controller "/1(pitch angle) -> [Beta], Wind Turbine/2(Pitch angle (deg))
  Relational Operator/1 -> [PWM1], Logical Operator4/1
  Gain2/1 -> Sum6/2
  [wt] -> dq0 to abc/2
  "Power (3ph, Instantaneous)"/1 -> Scope5/1
  dq0 to abc/1 -> Demux3/1
  [VQ] -> Sum7/2
  Demux/1 -> [VD]
  Integrator/1 -> Alpha-Beta-Zero to dq1/2, [wt]
  Logical Operator3/1 -> [PWM4]
  Constant2/1 -> Sum/2
  [alphabeta] -> Alpha-Beta-Zero to dq1/1
  Product1/1 -> Mux/2
  Gain1/1 -> Product/1
  Demux3/2 -> Relational Operator1/1
  Repeating Sequence2/1 -> Rate Limiter1/1
  Wr/1 -> con to (P.U)/2, Product3/2
  [VDC] -> Scope6/1
  Bus Selector/2 -> Scope8/2, con to (P.U)/1  "<Rotor speed wm (rad/s)>"
  Demux/2 -> [VQ]
  Relational Operator2/1 -> [PWM5], Logical Operator5/1
  Demux1/3 -> ?
  [VD] -> Sum4/2
  Demux1/1 -> [ID]
  Alpha-Beta-Zero to dq0/1 -> Demux/1
  [PWM6] -> IGBT/Diode5/1
  Logical Operator4/1 -> [PWM2]
  Constant4/1 -> Sum5/1
  Sum4/1 -> Gain1/1
  Sum2/1 -> PID Controller2/1
  Sum3/1 -> Sum4/1
  Pac/1(Out1) -> Scope10/1, [Pmeas]
  PID Controller3/1 -> Sum6/1
  [PWM4] -> IGBT/Diode4/1
  Repeating Sequence/1 -> Relational Operator2/2, Relational Operator1/2, Relational Operator/2
  PID Controller2/1 -> Sum3/1
  Demux2/3 -> ?
  [PWM5] -> IGBT/Diode2/1
  Demux3/3 -> Relational Operator2/1
  [IQ] -> Sum5/2
  [Iabc] -> "Power (3ph, Instantaneous)"/2, Scope3/1
  [Pmeas] -> Scope9/4
  [PWM2] -> IGBT/Diode3/1
  [PWM1] -> IGBT/Diode/1
  Product/1 -> Mux/1
  [Vabc3] -> abc to Alpha-Beta-Zero/1
  Voltage Measurement2/1 -> Scope8/4, Pac/1(In1)  "VL_L"
  abc to Alpha-Beta-Zero/1 -> Alpha-Beta-Zero to dq0/1, [alphabeta]
  abc to dq0/1 -> Demux1/1
  PID Controller/1 -> Integrator/1
  "Power (3ph, Instantaneous)"/2 -> Scope4/1
  Iout/1 -> Idc out/1
  Sum5/1 -> PID Controller3/1
  Sum/1 -> PID Controller/1
  Vdc out/1 -> Product4/2, Vout./1, [Vdc_out]
  PID Controller1/1 -> Sum2/1
  [wt] -> abc to dq0/2
  [PWM3] -> IGBT/Diode1/1
  RMS/1 -> Display/1
  Unit Delay2/1 -> Demux5/1
  Relay/1(Out1) -> Three-Phase Breaker/1
  Demux5/3 -> Relay/3(In3)
  Demux5/1 -> Relay/1(In1)
  Demux5/2 -> Relay/2(In2)
  Three-Phase V-I Measurement3/2 -> Scope/2, RMS/1, Unit Delay2/1
  Three-Phase V-I Measurement3/1 -> Scope/1
  connections:
  Current Measurement/RConn1 -- Universal Bridge/LConn1
  Universal Bridge/LConn3 -- Three-Phase V-I Measurement/RConn3
  Series RLC Branch11/LConn1 -- Idc/RConn1 -- Series RLC Branch9/RConn1
  PMSM/LConn3 -- Three-Phase V-I Measurement/LConn3
  Three-Phase V-I Measurement2/LConn1 -- Three-Phase Transformer (Two Windings)/LConn1
  Three-Phase V-I Measurement3/LConn3 -- Three-Phase Transformer (Two Windings)/RConn3
  Three-Phase V-I Measurement3/LConn2 -- Three-Phase Transformer (Two Windings)/RConn2
  Three-Phase V-I Measurement3/LConn1 -- Three-Phase Transformer (Two Windings)/RConn1
  Three-Phase V-I Measurement/LConn2 -- PMSM/LConn2
  Three-Phase V-I Measurement/RConn2 -- Voltage Measurement2/LConn2 -- Universal Bridge/LConn2
  Three-Phase V-I Measurement/LConn1 -- PMSM/LConn1
  Current Measurement/LConn1 -- Three-Phase V-I Measurement/RConn1 -- Voltage Measurement2/LConn1
  Diode1/LConn1 -- Series RLC Branch9/LConn1 -- IGBT/Diode6/LConn1
  Three-Phase V-I Measurement2/LConn3 -- Three-Phase Transformer (Two Windings)/LConn3
  Series RLC Branch6/LConn1 -- Series RLC Branch3/LConn1 -- Series RLC Branch/RConn1
  Series RLC Branch7/LConn1 -- Series RLC Branch4/LConn1 -- Series RLC Branch1/RConn1
  Series RLC Branch5/RConn1 -- Three-Phase V-I Measurement2/RConn3
  Iout/RConn1 -- Vout/LConn1
  Series RLC Branch2/LConn1 -- Three-Phase V-I Measurement1/RConn3
  Three-Phase V-I Measurement2/LConn2 -- Three-Phase Transformer (Two Windings)/LConn2
  Vdc/LConn1 -- Idc/LConn1 -- Ci/LConn1 -- Universal Bridge/RConn1
  Series RLC Branch3/RConn1 -- Three-Phase V-I Measurement2/RConn1
  Series RLC Branch/LConn1 -- Three-Phase V-I Measurement1/RConn1
  Series RLC Branch7/RConn1 -- Series RLC Branch8/RConn1 -- Series RLC Branch6/RConn1
  IGBT/Diode4/LConn1 -- IGBT/Diode1/RConn1 -- Three-Phase V-I Measurement1/LConn2
  Series RLC Branch8/LConn1 -- Series RLC Branch5/LConn1 -- Series RLC Branch2/RConn1
  Series RLC Branch11/RConn1 -- Vdc/LConn2 -- Universal Bridge/RConn2 -- Ci/RConn1 -- IGBT/Diode6/RConn1 -- Series RLC Branch10/RConn1 -- Vout/LConn2 -- IGBT/Diode4/RConn1 -- IGBT/Diode5/RConn1 -- IGBT/Diode3/RConn1 -- Voltage Measurement/LConn2
  IGBT/Diode3/LConn1 -- Three-Phase V-I Measurement1/LConn1 -- IGBT/Diode/RConn1
  Series RLC Branch4/RConn1 -- Three-Phase V-I Measurement2/RConn2
  Series RLC Branch1/LConn1 -- Three-Phase V-I Measurement1/RConn2
  IGBT/Diode5/LConn1 -- IGBT/Diode2/RConn1 -- Three-Phase V-I Measurement1/LConn3
  Diode1/RConn1 -- Iout/LConn1 -- Voltage Measurement/LConn1 -- IGBT/Diode1/LConn1 -- IGBT/Diode2/LConn1 -- IGBT/Diode/LConn1 -- Series RLC Branch10/LConn1
  Three-Phase V-I Measurement3/RConn3 -- Three-Phase Breaker/RConn3
  Three-Phase V-I Measurement3/RConn2 -- Three-Phase Breaker/RConn2
  Three-Phase V-I Measurement3/RConn1 -- Three-Phase Breaker/RConn1
  Three-Phase Breaker/LConn1 -- Connection Port/RConn1
  Three-Phase Breaker/LConn2 -- Connection Port1/RConn1
  Three-Phase Breaker/LConn3 -- Connection Port2/RConn1

== system Smart_Grid_2/Wind_Farm 48KW/Wind_Turbine 1/Pac ==
  In1 : Inport
  In2 : Inport  Port=2
  >> KW : Gain  Gain=1/1000
  Gain1 : Gain  Gain=1.732
  Product3 : Product  Inputs=**
  RMS : spsRMSLib/RMS  TrueRMS=on  Freq=50  RMSInit=120  Ts=50e-6
  RMS1 : spsRMSLib/RMS  TrueRMS=on  Freq=50  RMSInit=120  Ts=50e-6
  sqrt(3) : Gain  Gain=1.732
  Out1 : Outport
  wires:
  RMS/1 -> Gain1/1
  RMS1/1 -> Product3/2
  Gain1/1 -> Product3/1
  sqrt(3)/1 -> >> KW/1
  Product3/1 -> sqrt(3)/1
  In2/1 -> RMS1/1
  >> KW/1 -> Out1/1
  In1/1 -> RMS/1

== system Smart_Grid_2/Wind_Farm 48KW/Wind_Turbine 1/Pitch angle controller  ==
  Pmeas : Inport
  >p.u : Gain  Gain=1/12.343
  PID Controller : slpidlib/PID Controller  Controller=PI  Form=Parallel  TimeDomain=Discrete-time  UseExternalTs=off  SampleTime=-1  IntegratorMethod=Forward Euler  FilterMethod=Forward Euler  ControllerParametersSource=internal  P=0.001  I=0.02  UseKiTs=off  D=0  UseExternalDerivativeSource=off  N=100  UseFilter=on  TunerSelectOption=Transfer Function Based (PID Tuner App)  InitialConditionSource=internal  InitialConditionForIntegrator=0  InitialConditionForFilter=0  DifferentiatorICPrevScaledInput=0  ExternalReset=none  TrackingMode=off  Kt=1  LimitOutput=off  SatLimitsSource=internal  UpperSaturationLimit=inf  LowerSaturationLimit=-inf  LinearizeAsGain=on  AntiWindupMode=none  Kb=1  LimitIntegrator=off  UpperIntegratorSaturationLimit=inf  LowerIntegratorSaturationLimit=-inf  POutMin=[]  POutMax=[]  IOutMin=[]  IOutMax=[]  DOutMin=[]  DOutMax=[]  NOutMin=[]  NOutMax=[]  SumOutMin=[]  SumOutMax=[]  SaturationOutMin=[]  SaturationOutMax=[]  PParamMin=[]  PParamMax=[]  IParamMin=[]  IParamMax=[]  DParamMin=[]  DParamMax=[]  NParamMin=[]  NParamMax=[]  KbParamMin=[]  KbParamMax=[]  KtParamMin=[]  KtParamMax=[]  KbOutMin=[]  KbOutMax=[]  KtOutMin=[]  KtOutMax=[]  IntegratorOutMin=[]  IntegratorOutMax=[]  FilterOutMin=[]  FilterOutMax=[]  SumI1OutMin=[]  SumI1OutMax=[]  SumI2OutMin=[]  SumI2OutMax=[]  SumI3OutMin=[]  SumI3OutMax=[]  SumI4OutMin=[]  SumI4OutMax=[]  SumDOutMin=[]  SumDOutMax=[]  DifferentiatorOutMin=[]  DifferentiatorOutMax=[]  FilterDiffOutCoefMin=[]  FilterDiffOutCoefMax=[]  ReciprocalOutMin=[]  ReciprocalOutMax=[]  SumDenOutMin=[]  SumDenOutMax=[]  SumNumOutMin=[]  SumNumOutMax=[]  DivideOutMin=[]  DivideOutMax=[]  UdiffTsProdOutMin=[]  UdiffTsProdOutMax=[]  NTsProdOutMin=[]  NTsProdOutMax=[]  UintegralTsProdOutMin=[]  UintegralTsProdOutMax=[]  UngainTsProdOutMin=[]  UngainTsProdOutMax=[]  ClampingZeroOutDataTypeStr=Inherit: Inherit via back propagation  ClampingZeroOutMin=[]  ClampingZeroOutMax=[]  FilterDenConstantOutDataTypeStr=Inherit: Inherit via back propagation  FilterDenConstantOutMin=[]  FilterDenConstantOutMax=[]  PCopyOutDataTypeStr=Inherit: Inherit via back propagation  PCopyOutMin=[]  PCopyOutMax=[]  NCopyOutDataTypeStr=Inherit: Inherit via back propagation  NCopyOutMin=[]  NCopyOutMax=[]  IntegratorContinuousStateAttributes=''  IntegratorStateMustResolveToSignalObject=off  IntegratorRTWStateStorageClass=Auto  FilterContinuousStateAttributes=''  FilterStateMustResolveToSignalObject=off  FilterRTWStateStorageClass=Auto  ParallelPVariant=InternalParameters  IdealPVariant=Disabled  IVariant=InternalParameters  DVariant=Disabled  IntegratorVariant=Discrete  SatVariant=Disabled  AWVariant=Passthrough  PCopyVariant=Disabled  TRVariant=Disabled  FdbkBlocksVariant=Forward  IdealPFdbkVariant=Disabled  SatFdbkVariant=Disabled  DerivativeFilterVariant=Disabled  NVariant=Disabled  NCopyVariant=Disabled_SignalSpec  FilterICVariant=Disabled  IntegratorICVariant=InternalICs  ExternalResetVariant=Disabled  TRSumVariant=Passthrough  SumFdbkVariant=Disabled  SumVariant=Sum_PI  TsampFilterVariant=InternalTs  TsampNgainVariant=Passthrough  TsampIntegralVariant=Disabled_SignalSpec  ExternalSaturationOutDataTypeStr=Inherit: Same as second input  DerivativeSourceVariant=Disabled  PreIntVariant=InternalPreInt
  Pmech/Pnom : Constant  Value=12300/(12300*0.9)
  Rate Limiter : RateLimiter  RisingSlewLimit=+2  FallingSlewLimit=-2  SampleTimeMode=inherited
  Saturation : Saturate  UpperLimit=45  LowerLimit=0
  Sum : Sum  Inputs=|+-
  pitch angle : Outport
  wires:
  >p.u/1 -> Sum/1
  Pmeas/1 -> >p.u/1
  Sum/1 -> PID Controller/1
  PID Controller/1 -> Saturation/1
  Saturation/1 -> Rate Limiter/1
  Rate Limiter/1 -> pitch angle/1
  Pmech/Pnom/1 -> Sum/2

== system Smart_Grid_2/Wind_Farm 48KW/Wind_Turbine 1/Relay ==
  In1 : Inport
  In2 : Inport  Port=2
  In3 : Inport  Port=3
  Constant4 : Constant  Value=12
  Constant5 : Constant  Value=0
  Data Type Conversion : DataTypeConversion  OutDataTypeStr=double  SaturateOnIntegerOverflow=off  RndMeth=Floor
  Logical Operator1 : Logic  Inputs=3  AllPortsSameDT=off  OutDataTypeStr=boolean
  RMS : spsRMSLib/RMS  TrueRMS=on  Freq=50  RMSInit=0  Ts=0.001
  RMS1 : spsRMSLib/RMS  TrueRMS=on  Freq=50  RMSInit=0  Ts=0.001
  RMS2 : spsRMSLib/RMS  TrueRMS=on  Freq=50  RMSInit=0  Ts=0.001
  Relational Operator : RelationalOperator  Operator=>  OutDataTypeStr=boolean  RndMeth=Simplest  InputSameDT=off
  Relational Operator1 : RelationalOperator  Operator=>  OutDataTypeStr=boolean  RndMeth=Simplest  InputSameDT=off
  Relational Operator2 : RelationalOperator  Operator=>  OutDataTypeStr=boolean  RndMeth=Simplest  InputSameDT=off
  Set-Reset Flip-Flop : eeGeneralControl/Set-Reset Flip-Flop  LabelModeActiveChoice=Discrete  UndefState=Set  Q0=0  Ts=0.001
  Set-Reset Flip-Flop1 : eeGeneralControl/Set-Reset Flip-Flop  LabelModeActiveChoice=Discrete  UndefState=Set  Q0=0  Ts=0.001
  Set-Reset Flip-Flop2 : eeGeneralControl/Set-Reset Flip-Flop  LabelModeActiveChoice=Discrete  UndefState=Reset  Q0=0  Ts=0.001
  Terminator1 : Terminator
  Terminator2 : Terminator
  Terminator3 : Terminator
  Out1 : Outport
  wires:
  In2/1 -> RMS1/1
  Relational Operator1/1 -> Set-Reset Flip-Flop2/1
  Constant4/1 -> Relational Operator/2, Relational Operator1/2, Relational Operator2/2
  Constant5/1 -> Set-Reset Flip-Flop1/2, Set-Reset Flip-Flop2/2, Set-Reset Flip-Flop/2
  Logical Operator1/1 -> Data Type Conversion/1
  Data Type Conversion/1 -> Out1/1
  In3/1 -> RMS2/1
  In1/1 -> RMS/1
  RMS1/1 -> Relational Operator1/1
  RMS2/1 -> Relational Operator2/1
  RMS/1 -> Relational Operator/1
  Relational Operator2/1 -> Set-Reset Flip-Flop/1
  Relational Operator/1 -> Set-Reset Flip-Flop1/1
  Set-Reset Flip-Flop/2 -> Logical Operator1/3
  Set-Reset Flip-Flop2/2 -> Logical Operator1/2
  Set-Reset Flip-Flop1/2 -> Logical Operator1/1
  Set-Reset Flip-Flop2/1 -> Terminator1/1
  Set-Reset Flip-Flop/1 -> Terminator3/1
  Set-Reset Flip-Flop1/1 -> Terminator2/1

== system Smart_Grid_2/Wind_Farm 48KW/Wind_Turbine 1/Wind Turbine ==
  Generator speed (pu) : Inport
  Pitch angle (deg) : Inport  Port=2
  Wind speed (m/s) : Inport  Port=3
  1/cp_nom : Gain  Gain=1/cp_nom  SaturateOnIntegerOverflow=on  OutDataTypeStr=Inherit: Same as input  ParamDataTypeStr=Inherit: Same as input
  1/wind_base : Gain  Gain=1/wind_base  SaturateOnIntegerOverflow=on  OutDataTypeStr=Inherit: Same as input  ParamDataTypeStr=Inherit: Same as input
  Avoid division by zero : Saturate  UpperLimit=1e6  LowerLimit=1e-6
  "Avoid division by zero " : Saturate  UpperLimit=1e6  LowerLimit=1e-6
  Gain : Gain  Gain=-1  SaturateOnIntegerOverflow=on  OutDataTypeStr=Inherit: Same as input  ParamDataTypeStr=Inherit: Same as input
  Product : Product  Inputs=/*  SaturateOnIntegerOverflow=on  OutDataTypeStr=Inherit: Same as first input
  "Product " : Product  SaturateOnIntegerOverflow=on  OutDataTypeStr=Inherit: Same as first input
  Product2 : Product  Inputs=*/  InputSameDT=on  SaturateOnIntegerOverflow=on  OutDataTypeStr=Inherit: Same as first input
  Saturation1 : Saturate  UpperLimit=inf  LowerLimit=1e-6
  cp(lambda,beta) : Subsystem
  lambda_nom : Gain  Gain=lambda_nom  SaturateOnIntegerOverflow=on  OutDataTypeStr=Inherit: Same as input  ParamDataTypeStr=Inherit: Same as input
  pu->pu : Gain  Gain=P_wind_base*Pnom/Pelec_base  SaturateOnIntegerOverflow=on  OutDataTypeStr=Inherit: Same as input  ParamDataTypeStr=Inherit: Same as input
  "pu->pu " : Gain  Gain=1/speed_nom  SaturateOnIntegerOverflow=on  OutDataTypeStr=Inherit: Same as input  ParamDataTypeStr=Inherit: Same as input
  wind_speed^3 : Fcn  Expr=u(1)^3
  Tm (pu) : Outport  VectorParamsAs1DForOutWhenUnconnected=off
  Cp : Outport  Port=2  VectorParamsAs1DForOutWhenUnconnected=off
  wires:
  "pu->pu "/1 -> Product/2
  "Avoid division by zero "/1 -> Product/1
  1/wind_base/1 -> "Avoid division by zero "/1, wind_speed^3/1  "wind_speed_pu"
  Product/1 -> lambda_nom/1  "lambda_pu"
  Saturation1/1 -> cp(lambda,beta)/1(lambda)
  1/cp_nom/1 -> "Product "/2  "cp_pu"
  lambda_nom/1 -> Saturation1/1  "lambda"
  "Product "/1 -> pu->pu/1  "Pm_pu"
  Generator speed (pu)/1 -> "pu->pu "/1, Avoid division by zero/1
  Gain/1 -> Tm (pu)/1
  Wind speed (m/s)/1 -> 1/wind_base/1
  Avoid division by zero/1 -> Product2/2
  Product2/1 -> Gain/1
  wind_speed^3/1 -> "Product "/1  "Pwind_pu"
  cp(lambda,beta)/1(cp) -> Cp/1, 1/cp_nom/1
  pu->pu/1 -> Product2/1
  Pitch angle (deg)/1 -> cp(lambda,beta)/2(beta)

== system Smart_Grid_2/Wind_Farm 48KW/Wind_Turbine 2/Pac ==
  In1 : Inport
  In2 : Inport  Port=2
  >> KW : Gain  Gain=1/1000
  Gain1 : Gain  Gain=1.732
  Product3 : Product  Inputs=**
  RMS : spsRMSLib/RMS  TrueRMS=on  Freq=50  RMSInit=120  Ts=50e-6
  RMS1 : spsRMSLib/RMS  TrueRMS=on  Freq=50  RMSInit=120  Ts=50e-6
  sqrt(3) : Gain  Gain=1.732
  Out1 : Outport
  wires:
  In1/1 -> RMS/1
  >> KW/1 -> Out1/1
  In2/1 -> RMS1/1
  Product3/1 -> sqrt(3)/1
  sqrt(3)/1 -> >> KW/1
  Gain1/1 -> Product3/1
  RMS1/1 -> Product3/2
  RMS/1 -> Gain1/1
